simulink model "battery_phfb_inv_single_phase"  (R2024b)
settings: Solver=ode1be  StartTime=0.0  StopTime=simlength  FixedStep=ts_sim  MaxStep=ts_sim
undefined symbols (not defined in the file): Adrso, Aresd, Bresd, Cresd, Crso, dead_time, DThs_init, fPWM_INV, fPWM_ZVS, frequency_grid, I_FS, Iout_dc_nom, ki_i_inv, ki_i_zvs, ki_pll, ki_v_inv, ki_v_zvs, kp_i_inv, kp_i_zvs, kp_pll, kp_v_inv, kp_v_zvs, Ldrso, LFu_dc, magnitude, n1, number_of_cells, Q, q1kalman, q1Kalman, q2kalman, q2Kalman, q3Kalman, RCFu_dc, Rkalman, rKalman, RLFu_dc, Rload, Tambient, tc, ts_inv, ts_zvs, tsample, v1_trafo, v2_trafo, V_FS, Vout_dc_nom, w, weigth
libraries: fl_lib x207, nesl_utility x105, ee_lib x26, cstblocks x7, single_phase_transformer_lib x4, lithium_ion_cell_lib x1, simulink x1
(part 2 of 8)

== system battery_phfb_inv_single_phase/inverter_modA/single phase inverter/HBridgeIdeal ==
  gate_commands : Inport
  Bus Selector : BusSelector  OutputSignals=gate_cmd_Q1 (signal 1),gate_cmd_Q2 (signal 2),gate_cmd_Q1 (signal 3),gate_cmd_Q2 (signal 4)
  Simulink-PS Converter{,1..3} (4 alike) : nesl_utility/Simulink-PS Converter  PhysicalDomain=network_engine_domain  SubClassName=ps_input  LeftPortType=input  RightPortType=output  PseudoPeriodic=off  Frequencies=[]  NoiseDistribution=none  NoiseParameters=[]  Unit=1  AffineConversion=on  FilteringAndDerivatives=provide  SimscapeFilterOrder=1  InputFilterTimeConstant=0.001  UdotUserProvided=0
  switch_1 : Subsystem
      settings: PortSchema="{\"entries\":[{\"content\":{\"sides\":[{\"content\":{\"connectorIds\":[\"LConn1\"]},\"type\":\"ConnectorPlacement.EquallySpacedRectSide\",\"uuid\":\"9277da8d-d460-43e6-8478-dd662f15d226\"},{\"content\":{\"connectorIds\":[],\"side\":\"RIGHT\"},\"type\":\"ConnectorPlacement.EquallySpacedRectSide\",\"uuid\":\"a7ece396-f1d9-4f4f-a05b-db1fc65d6e1d\"},{\"content\":{\"connectorIds\":[\"LConn2\"],\"side\":\"TOP\"},\"type\":\"ConnectorPlacement.EquallySpacedRectSide\",\"uuid\":\"fdd70777-e9cf-4317-afb6-cae87f75d5b0\"},{\"content\":{\"connectorIds\":[\"RConn1\"],\"side\":\"BOTTOM\"},\"type\":\"ConnectorPlacement.EquallySpacedRectSide\",\"uuid\":\"2353ed68-b1a1-4775-9ca9-31e268d5443b\"}]},\"type\":\"ConnectorPlacement.EquallySpacedConnector\",\"uuid\":\"d5479f4c-4e65-4791-adcb-73df11f88590\"}],\"packageUris\":[\"http://schema.mathworks.com/mf0/Connector/R2020b\"],\"version\":\"1.0\"}"
  switch_2 : Subsystem
      settings: PortSchema="{\"entries\":[{\"content\":{\"sides\":[{\"content\":{\"connectorIds\":[\"LConn1\"]},\"type\":\"ConnectorPlacement.EquallySpacedRectSide\",\"uuid\":\"9277da8d-d460-43e6-8478-dd662f15d226\"},{\"content\":{\"connectorIds\":[],\"side\":\"RIGHT\"},\"type\":\"ConnectorPlacement.EquallySpacedRectSide\",\"uuid\":\"a7ece396-f1d9-4f4f-a05b-db1fc65d6e1d\"},{\"content\":{\"connectorIds\":[\"LConn2\"],\"side\":\"TOP\"},\"type\":\"ConnectorPlacement.EquallySpacedRectSide\",\"uuid\":\"fdd70777-e9cf-4317-afb6-cae87f75d5b0\"},{\"content\":{\"connectorIds\":[\"RConn1\"],\"side\":\"BOTTOM\"},\"type\":\"ConnectorPlacement.EquallySpacedRectSide\",\"uuid\":\"2353ed68-b1a1-4775-9ca9-31e268d5443b\"}]},\"type\":\"ConnectorPlacement.EquallySpacedConnector\",\"uuid\":\"d5479f4c-4e65-4791-adcb-73df11f88590\"}],\"packageUris\":[\"http://schema.mathworks.com/mf0/Connector/R2020b\"],\"version\":\"1.0\"}"
  switch_3 : Subsystem
      settings: PortSchema="{\"entries\":[{\"content\":{\"sides\":[{\"content\":{\"connectorIds\":[\"LConn1\"]},\"type\":\"ConnectorPlacement.EquallySpacedRectSide\",\"uuid\":\"9277da8d-d460-43e6-8478-dd662f15d226\"},{\"content\":{\"connectorIds\":[],\"side\":\"RIGHT\"},\"type\":\"ConnectorPlacement.EquallySpacedRectSide\",\"uuid\":\"a7ece396-f1d9-4f4f-a05b-db1fc65d6e1d\"},{\"content\":{\"connectorIds\":[\"LConn2\"],\"side\":\"TOP\"},\"type\":\"ConnectorPlacement.EquallySpacedRectSide\",\"uuid\":\"fdd70777-e9cf-4317-afb6-cae87f75d5b0\"},{\"content\":{\"connectorIds\":[\"RConn1\"],\"side\":\"BOTTOM\"},\"type\":\"ConnectorPlacement.EquallySpacedRectSide\",\"uuid\":\"2353ed68-b1a1-4775-9ca9-31e268d5443b\"}]},\"type\":\"ConnectorPlacement.EquallySpacedConnector\",\"uuid\":\"d5479f4c-4e65-4791-adcb-73df11f88590\"}],\"packageUris\":[\"http://schema.mathworks.com/mf0/Connector/R2020b\"],\"version\":\"1.0\"}"
  switch_4 : Subsystem
      settings: PortSchema="{\"entries\":[{\"content\":{\"sides\":[{\"content\":{\"connectorIds\":[\"LConn1\"]},\"type\":\"ConnectorPlacement.EquallySpacedRectSide\",\"uuid\":\"9277da8d-d460-43e6-8478-dd662f15d226\"},{\"content\":{\"connectorIds\":[],\"side\":\"RIGHT\"},\"type\":\"ConnectorPlacement.EquallySpacedRectSide\",\"uuid\":\"a7ece396-f1d9-4f4f-a05b-db1fc65d6e1d\"},{\"content\":{\"connectorIds\":[\"LConn2\"],\"side\":\"TOP\"},\"type\":\"ConnectorPlacement.EquallySpacedRectSide\",\"uuid\":\"fdd70777-e9cf-4317-afb6-cae87f75d5b0\"},{\"content\":{\"connectorIds\":[\"RConn1\"],\"side\":\"BOTTOM\"},\"type\":\"ConnectorPlacement.EquallySpacedRectSide\",\"uuid\":\"2353ed68-b1a1-4775-9ca9-31e268d5443b\"}]},\"type\":\"ConnectorPlacement.EquallySpacedConnector\",\"uuid\":\"d5479f4c-4e65-4791-adcb-73df11f88590\"}],\"packageUris\":[\"http://schema.mathworks.com/mf0/Connector/R2020b\"],\"version\":\"1.0\"}"
  C : PMIOPort  Side=Left
  E : PMIOPort  Port=2  Side=Right
  C1 : PMIOPort  Port=3  Side=Right
  E1 : PMIOPort  Port=4  Side=Left
  wires:
  [gate_Q3] -> Simulink-PS Converter2/1
  Bus Selector/2 -> [gate_Q2]  "<gate_cmd_Q2 (signal 2)>"
  Bus Selector/1 -> [gate_Q1]  "<gate_cmd_Q1 (signal 1)>"
  Bus Selector/3 -> [gate_Q3]  "<gate_cmd_Q1 (signal 3)>"
  [gate_Q4] -> Simulink-PS Converter3/1
  [gate_Q2] -> Simulink-PS Converter1/1
  [gate_Q1] -> Simulink-PS Converter/1
  Bus Selector/4 -> [gate_Q4]  "<gate_cmd_Q2 (signal 4)>"
  gate_commands/1 -> Bus Selector/1
  connections:
  switch_1/LConn1 -- Simulink-PS Converter/RConn1
  switch_3/LConn2 -- C/RConn1 -- switch_1/LConn2
  switch_4/RConn1 -- E1/RConn1 -- switch_2/RConn1
  switch_2/LConn2 -- E/RConn1 -- switch_1/RConn1
  switch_3/LConn1 -- Simulink-PS Converter2/RConn1
  switch_3/RConn1 -- C1/RConn1 -- switch_4/LConn2
  switch_2/LConn1 -- Simulink-PS Converter1/RConn1
  switch_4/LConn1 -- Simulink-PS Converter3/RConn1

== system battery_phfb_inv_single_phase/inverter_modA/single phase inverter/HBridgeMosfet ==
  gate_commands : Inport
  Bus Selector : BusSelector  OutputSignals=gate_cmd_Q1,gate_cmd_Q2,gate_cmd_Q3,gate_cmd_Q4
  Simulink-PS Converter{,1..3} (4 alike) : nesl_utility/Simulink-PS Converter  PhysicalDomain=network_engine_domain  SubClassName=ps_input  LeftPortType=input  RightPortType=output  PseudoPeriodic=off  Frequencies=[]  NoiseDistribution=none  NoiseParameters=[]  Unit=V  AffineConversion=off  FilteringAndDerivatives=provide  SimscapeFilterOrder=1  InputFilterTimeConstant=0.001  UdotUserProvided=0
  mosfet_1 : Subsystem
      settings: PortSchema="{\"entries\":[{\"content\":{\"sides\":[{\"content\":{\"connectorIds\":[\"LConn1\"]},\"type\":\"ConnectorPlacement.EquallySpacedRectSide\",\"uuid\":\"9277da8d-d460-43e6-8478-dd662f15d226\"},{\"content\":{\"connectorIds\":[],\"side\":\"RIGHT\"},\"type\":\"ConnectorPlacement.EquallySpacedRectSide\",\"uuid\":\"a7ece396-f1d9-4f4f-a05b-db1fc65d6e1d\"},{\"content\":{\"connectorIds\":[\"LConn2\"],\"side\":\"TOP\"},\"type\":\"ConnectorPlacement.EquallySpacedRectSide\",\"uuid\":\"fdd70777-e9cf-4317-afb6-cae87f75d5b0\"},{\"content\":{\"connectorIds\":[\"RConn1\"],\"side\":\"BOTTOM\"},\"type\":\"ConnectorPlacement.EquallySpacedRectSide\",\"uuid\":\"2353ed68-b1a1-4775-9ca9-31e268d5443b\"}]},\"type\":\"ConnectorPlacement.EquallySpacedConnector\",\"uuid\":\"d5479f4c-4e65-4791-adcb-73df11f88590\"}],\"packageUris\":[\"http://schema.mathworks.com/mf0/Connector/R2020b\"],\"version\":\"1.0\"}"
  mosfet_2 : Subsystem
      settings: PortSchema="{\"entries\":[{\"content\":{\"sides\":[{\"content\":{\"connectorIds\":[\"LConn1\"]},\"type\":\"ConnectorPlacement.EquallySpacedRectSide\",\"uuid\":\"9277da8d-d460-43e6-8478-dd662f15d226\"},{\"content\":{\"connectorIds\":[],\"side\":\"RIGHT\"},\"type\":\"ConnectorPlacement.EquallySpacedRectSide\",\"uuid\":\"a7ece396-f1d9-4f4f-a05b-db1fc65d6e1d\"},{\"content\":{\"connectorIds\":[\"LConn2\"],\"side\":\"TOP\"},\"type\":\"ConnectorPlacement.EquallySpacedRectSide\",\"uuid\":\"fdd70777-e9cf-4317-afb6-cae87f75d5b0\"},{\"content\":{\"connectorIds\":[\"RConn1\"],\"side\":\"BOTTOM\"},\"type\":\"ConnectorPlacement.EquallySpacedRectSide\",\"uuid\":\"2353ed68-b1a1-4775-9ca9-31e268d5443b\"}]},\"type\":\"ConnectorPlacement.EquallySpacedConnector\",\"uuid\":\"d5479f4c-4e65-4791-adcb-73df11f88590\"}],\"packageUris\":[\"http://schema.mathworks.com/mf0/Connector/R2020b\"],\"version\":\"1.0\"}"
  mosfet_3 : Subsystem
      settings: PortSchema="{\"entries\":[{\"content\":{\"sides\":[{\"content\":{\"connectorIds\":[\"LConn1\"]},\"type\":\"ConnectorPlacement.EquallySpacedRectSide\",\"uuid\":\"9277da8d-d460-43e6-8478-dd662f15d226\"},{\"content\":{\"connectorIds\":[],\"side\":\"RIGHT\"},\"type\":\"ConnectorPlacement.EquallySpacedRectSide\",\"uuid\":\"a7ece396-f1d9-4f4f-a05b-db1fc65d6e1d\"},{\"content\":{\"connectorIds\":[\"LConn2\"],\"side\":\"TOP\"},\"type\":\"ConnectorPlacement.EquallySpacedRectSide\",\"uuid\":\"fdd70777-e9cf-4317-afb6-cae87f75d5b0\"},{\"content\":{\"connectorIds\":[\"RConn1\"],\"side\":\"BOTTOM\"},\"type\":\"ConnectorPlacement.EquallySpacedRectSide\",\"uuid\":\"2353ed68-b1a1-4775-9ca9-31e268d5443b\"}]},\"type\":\"ConnectorPlacement.EquallySpacedConnector\",\"uuid\":\"d5479f4c-4e65-4791-adcb-73df11f88590\"}],\"packageUris\":[\"http://schema.mathworks.com/mf0/Connector/R2020b\"],\"version\":\"1.0\"}"
  mosfet_4 : Subsystem
      settings: PortSchema="{\"entries\":[{\"content\":{\"sides\":[{\"content\":{\"connectorIds\":[\"LConn1\"]},\"type\":\"ConnectorPlacement.EquallySpacedRectSide\",\"uuid\":\"9277da8d-d460-43e6-8478-dd662f15d226\"},{\"content\":{\"connectorIds\":[],\"side\":\"RIGHT\"},\"type\":\"ConnectorPlacement.EquallySpacedRectSide\",\"uuid\":\"a7ece396-f1d9-4f4f-a05b-db1fc65d6e1d\"},{\"content\":{\"connectorIds\":[\"LConn2\"],\"side\":\"TOP\"},\"type\":\"ConnectorPlacement.EquallySpacedRectSide\",\"uuid\":\"fdd70777-e9cf-4317-afb6-cae87f75d5b0\"},{\"content\":{\"connectorIds\":[\"RConn1\"],\"side\":\"BOTTOM\"},\"type\":\"ConnectorPlacement.EquallySpacedRectSide\",\"uuid\":\"2353ed68-b1a1-4775-9ca9-31e268d5443b\"}]},\"type\":\"ConnectorPlacement.EquallySpacedConnector\",\"uuid\":\"d5479f4c-4e65-4791-adcb-73df11f88590\"}],\"packageUris\":[\"http://schema.mathworks.com/mf0/Connector/R2020b\"],\"version\":\"1.0\"}"
  C : PMIOPort  Side=Left
  E : PMIOPort  Port=2  Side=Right
  C1 : PMIOPort  Port=3  Side=Right
  E1 : PMIOPort  Port=4  Side=Left
  wires:
  [gate_Q3] -> Simulink-PS Converter2/1
  Bus Selector/2 -> [gate_Q2]  "<gate_cmd_Q2>"
  Bus Selector/1 -> [gate_Q1]  "<gate_cmd_Q1>"
  Bus Selector/3 -> [gate_Q3]  "<gate_cmd_Q3>"
  [gate_Q4] -> Simulink-PS Converter3/1
  [gate_Q2] -> Simulink-PS Converter1/1
  [gate_Q1] -> Simulink-PS Converter/1
  Bus Selector/4 -> [gate_Q4]  "<gate_cmd_Q4>"
  gate_commands/1 -> Bus Selector/1
  connections:
  mosfet_1/LConn1 -- Simulink-PS Converter/RConn1
  C/RConn1 -- mosfet_3/LConn2 -- mosfet_1/LConn2
  E1/RConn1 -- mosfet_4/RConn1 -- mosfet_2/RConn1
  E/RConn1 -- mosfet_2/LConn2 -- mosfet_1/RConn1
  mosfet_3/LConn1 -- Simulink-PS Converter2/RConn1
  C1/RConn1 -- mosfet_4/LConn2 -- mosfet_3/RConn1
  mosfet_2/LConn1 -- Simulink-PS Converter1/RConn1
  mosfet_4/LConn1 -- Simulink-PS Converter3/RConn1

== system battery_phfb_inv_single_phase/inverter_modA/single phase inverter/HBridgeThermal ==
  gate_commands : Inport
  Bus Selector : BusSelector  OutputSignals=gate_cmd_Q1,gate_cmd_Q2,gate_cmd_Q3,gate_cmd_Q4
  Simulink-PS Converter{,1..3} (4 alike) : nesl_utility/Simulink-PS Converter  PhysicalDomain=network_engine_domain  SubClassName=ps_input  LeftPortType=input  RightPortType=output  PseudoPeriodic=off  Frequencies=[]  NoiseDistribution=none  NoiseParameters=[]  Unit=V  AffineConversion=off  FilteringAndDerivatives=provide  SimscapeFilterOrder=1  InputFilterTimeConstant=0.001  UdotUserProvided=0
  mosfet_thermal_1 : Subsystem
      settings: PortSchema="{\"entries\":[{\"content\":{\"sides\":[{\"content\":{\"connectorIds\":[\"LConn1\"]},\"type\":\"ConnectorPlacement.EquallySpacedRectSide\",\"uuid\":\"9277da8d-d460-43e6-8478-dd662f15d226\"},{\"content\":{\"connectorIds\":[],\"side\":\"RIGHT\"},\"type\":\"ConnectorPlacement.EquallySpacedRectSide\",\"uuid\":\"a7ece396-f1d9-4f4f-a05b-db1fc65d6e1d\"},{\"content\":{\"connectorIds\":[\"LConn2\"],\"side\":\"TOP\"},\"type\":\"ConnectorPlacement.EquallySpacedRectSide\",\"uuid\":\"fdd70777-e9cf-4317-afb6-cae87f75d5b0\"},{\"content\":{\"connectorIds\":[\"RConn1\"],\"side\":\"BOTTOM\"},\"type\":\"ConnectorPlacement.EquallySpacedRectSide\",\"uuid\":\"2353ed68-b1a1-4775-9ca9-31e268d5443b\"}]},\"type\":\"ConnectorPlacement.EquallySpacedConnector\",\"uuid\":\"d5479f4c-4e65-4791-adcb-73df11f88590\"}],\"packageUris\":[\"http://schema.mathworks.com/mf0/Connector/R2020b\"],\"version\":\"1.0\"}"
  mosfet_thermal_2 : Subsystem
      settings: PortSchema="{\"entries\":[{\"content\":{\"sides\":[{\"content\":{\"connectorIds\":[\"LConn1\"]},\"type\":\"ConnectorPlacement.EquallySpacedRectSide\",\"uuid\":\"9277da8d-d460-43e6-8478-dd662f15d226\"},{\"content\":{\"connectorIds\":[],\"side\":\"RIGHT\"},\"type\":\"ConnectorPlacement.EquallySpacedRectSide\",\"uuid\":\"a7ece396-f1d9-4f4f-a05b-db1fc65d6e1d\"},{\"content\":{\"connectorIds\":[\"LConn2\"],\"side\":\"TOP\"},\"type\":\"ConnectorPlacement.EquallySpacedRectSide\",\"uuid\":\"fdd70777-e9cf-4317-afb6-cae87f75d5b0\"},{\"content\":{\"connectorIds\":[\"RConn1\"],\"side\":\"BOTTOM\"},\"type\":\"ConnectorPlacement.EquallySpacedRectSide\",\"uuid\":\"2353ed68-b1a1-4775-9ca9-31e268d5443b\"}]},\"type\":\"ConnectorPlacement.EquallySpacedConnector\",\"uuid\":\"d5479f4c-4e65-4791-adcb-73df11f88590\"}],\"packageUris\":[\"http://schema.mathworks.com/mf0/Connector/R2020b\"],\"version\":\"1.0\"}"
  mosfet_thermal_3 : Subsystem
      settings: PortSchema="{\"entries\":[{\"content\":{\"sides\":[{\"content\":{\"connectorIds\":[\"LConn1\"]},\"type\":\"ConnectorPlacement.EquallySpacedRectSide\",\"uuid\":\"9277da8d-d460-43e6-8478-dd662f15d226\"},{\"content\":{\"connectorIds\":[],\"side\":\"RIGHT\"},\"type\":\"ConnectorPlacement.EquallySpacedRectSide\",\"uuid\":\"a7ece396-f1d9-4f4f-a05b-db1fc65d6e1d\"},{\"content\":{\"connectorIds\":[\"LConn2\"],\"side\":\"TOP\"},\"type\":\"ConnectorPlacement.EquallySpacedRectSide\",\"uuid\":\"fdd70777-e9cf-4317-afb6-cae87f75d5b0\"},{\"content\":{\"connectorIds\":[\"RConn1\"],\"side\":\"BOTTOM\"},\"type\":\"ConnectorPlacement.EquallySpacedRectSide\",\"uuid\":\"2353ed68-b1a1-4775-9ca9-31e268d5443b\"}]},\"type\":\"ConnectorPlacement.EquallySpacedConnector\",\"uuid\":\"d5479f4c-4e65-4791-adcb-73df11f88590\"}],\"packageUris\":[\"http://schema.mathworks.com/mf0/Connector/R2020b\"],\"version\":\"1.0\"}"
  mosfet_thermal_4 : Subsystem
      settings: PortSchema="{\"entries\":[{\"content\":{\"sides\":[{\"content\":{\"connectorIds\":[\"LConn1\"]},\"type\":\"ConnectorPlacement.EquallySpacedRectSide\",\"uuid\":\"9277da8d-d460-43e6-8478-dd662f15d226\"},{\"content\":{\"connectorIds\":[],\"side\":\"RIGHT\"},\"type\":\"ConnectorPlacement.EquallySpacedRectSide\",\"uuid\":\"a7ece396-f1d9-4f4f-a05b-db1fc65d6e1d\"},{\"content\":{\"connectorIds\":[\"LConn2\"],\"side\":\"TOP\"},\"type\":\"ConnectorPlacement.EquallySpacedRectSide\",\"uuid\":\"fdd70777-e9cf-4317-afb6-cae87f75d5b0\"},{\"content\":{\"connectorIds\":[\"RConn1\"],\"side\":\"BOTTOM\"},\"type\":\"ConnectorPlacement.EquallySpacedRectSide\",\"uuid\":\"2353ed68-b1a1-4775-9ca9-31e268d5443b\"}]},\"type\":\"ConnectorPlacement.EquallySpacedConnector\",\"uuid\":\"d5479f4c-4e65-4791-adcb-73df11f88590\"}],\"packageUris\":[\"http://schema.mathworks.com/mf0/Connector/R2020b\"],\"version\":\"1.0\"}"
  C : PMIOPort  Side=Left
  E : PMIOPort  Port=2  Side=Right
  C1 : PMIOPort  Port=3  Side=Right
  E1 : PMIOPort  Port=4  Side=Left
  wires:
  gate_commands/1 -> Bus Selector/1
  Bus Selector/4 -> [gate_Q4]  "<gate_cmd_Q4>"
  [gate_Q1] -> Simulink-PS Converter/1
  [gate_Q2] -> Simulink-PS Converter1/1
  [gate_Q4] -> Simulink-PS Converter3/1
  Bus Selector/3 -> [gate_Q3]  "<gate_cmd_Q3>"
  Bus Selector/1 -> [gate_Q1]  "<gate_cmd_Q1>"
  Bus Selector/2 -> [gate_Q2]  "<gate_cmd_Q2>"
  [gate_Q3] -> Simulink-PS Converter2/1
  connections:
  mosfet_thermal_4/LConn1 -- Simulink-PS Converter3/RConn1
  mosfet_thermal_2/LConn1 -- Simulink-PS Converter1/RConn1
  C1/RConn1 -- mosfet_thermal_4/LConn2 -- mosfet_thermal_3/RConn1
  mosfet_thermal_3/LConn1 -- Simulink-PS Converter2/RConn1
  E/RConn1 -- mosfet_thermal_1/RConn1 -- mosfet_thermal_2/LConn2
  E1/RConn1 -- mosfet_thermal_4/RConn1 -- mosfet_thermal_2/RConn1
  mosfet_thermal_1/LConn2 -- mosfet_thermal_3/LConn2 -- C/RConn1
  mosfet_thermal_1/LConn1 -- Simulink-PS Converter/RConn1

== system battery_phfb_inv_single_phase/inverter_modA/single phase inverter control/acquisition_and_scaling_current ==
  in : Inport
  1/Ti5 : Gain  Gain=1/I_FS  SaturateOnIntegerOverflow=on  OutDataTypeStr=Inherit: Same as input  ParamDataTypeStr=Inherit: Same as input
  Unit Delay4 : UnitDelay  SampleTime=ts_inv  HasFrameUpgradeWarning=on
  Zero-Order Hold1 : ZeroOrderHold  SampleTime=ts_inv
  out : Outport
  wires:
  in/1 -> Zero-Order Hold1/1
  1/Ti5/1 -> Unit Delay4/1
  Zero-Order Hold1/1 -> 1/Ti5/1
  Unit Delay4/1 -> out/1

== system battery_phfb_inv_single_phase/inverter_modA/single phase inverter control/acquisition_and_scaling_voltage ==
  in : Inport
  1/Ti1 : Gain  Gain=1/V_FS  SaturateOnIntegerOverflow=on  OutDataTypeStr=Inherit: Same as input  ParamDataTypeStr=Inherit: Same as input
  Unit Delay4 : UnitDelay  SampleTime=ts_inv  HasFrameUpgradeWarning=on
  Zero-Order Hold2 : ZeroOrderHold  SampleTime=ts_inv
  out : Outport
  wires:
  1/Ti1/1 -> Unit Delay4/1
  Zero-Order Hold2/1 -> 1/Ti1/1
  Unit Delay4/1 -> out/1
  in/1 -> Zero-Order Hold2/1

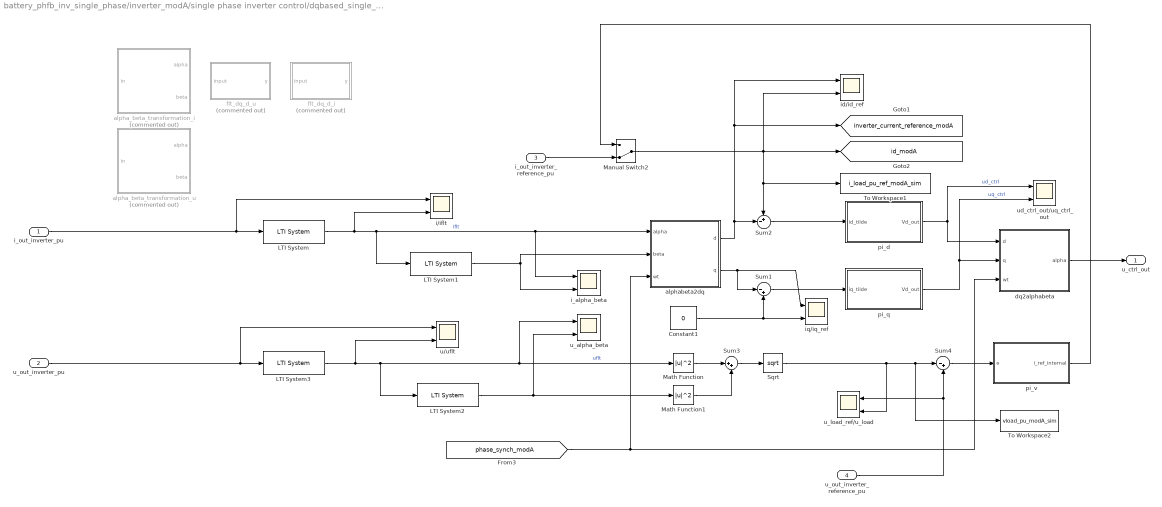
== system battery_phfb_inv_single_phase/inverter_modA/single phase inverter control/dqbased_single_phase_inverter_ctrl ==
  i_out_inverter_pu : Inport
  u_out_inverter_pu : Inport  Port=2
  i_out_inverter_reference_pu : Inport  Port=3
  u_out_inverter_reference_pu : Inport  Port=4
  Constant1 : Constant  Value=0
  LTI System : cstblocks/LTI System  sys=resd_tf  IC=[]  PadeOrder=0
  LTI System1 : cstblocks/LTI System  sys=flt_dq_d  IC=[]  PadeOrder=0
  LTI System2 : cstblocks/LTI System  sys=flt_dq_d  IC=[]  PadeOrder=0
  LTI System3 : cstblocks/LTI System  sys=resd_tf  IC=[]  PadeOrder=0
  Manual Switch2 : ManualSwitch  CurrentSetting=0
  Math Function : Math  Operator=magnitude^2
  Math Function1 : Math  Operator=magnitude^2
  Sqrt : Sqrt
  Sum1 : Sum  Inputs=|-+
  Sum2 : Sum  Inputs=+-|
  Sum3 : Sum  Inputs=|++
  Sum4 : Sum  Inputs=|-+
  To Workspace1 : ToWorkspace  VariableName=i_load_pu_ref_modA_sim  SampleTime=ts_inv
      settings: MaxDataPoints=Ns_inv
  To Workspace2 : ToWorkspace  VariableName=vload_pu_modA_sim  SampleTime=ts_inv
      settings: MaxDataPoints=Ns_inv
  alpha_beta_transformation_i : Subsystem  Commented=on
  alpha_beta_transformation_u : Subsystem  Commented=on
  alphabeta2dq : Subsystem
  dq2alphabeta : Subsystem
  flt_dq_d_i : MATLAB Function  Commented=on  TreatAsAtomicUnit=on  SystemSampleTime=ts_inv
  flt_dq_d_u : MATLAB Function  Commented=on  TreatAsAtomicUnit=on  SystemSampleTime=ts_inv
  i/iflt : Scope  NumInputPorts=2
  i_alpha_beta : Scope  NumInputPorts=2
  id/id_ref : Scope  NumInputPorts=2
  iq/iq_ref : Scope  NumInputPorts=2
  pi_d : Subsystem
  pi_q : Subsystem
  pi_v : Subsystem
  u/uflt : Scope  NumInputPorts=2
  u_alpha_beta : Scope  NumInputPorts=2
  u_load_ref/u_load : Scope  NumInputPorts=2
  ud_ctrl_out/uq_ctrl_out : Scope  NumInputPorts=2
  u_ctrl_out : Outport
  tag scope: id_modA=global, inverter_current_reference_modA=global
  wires:
  alphabeta2dq/1("d ") -> Sum2/2, id/id_ref/1, [inverter_current_reference_modA]
  Sqrt/1 -> u_load_ref/u_load/2, To Workspace2/1, Sum4/1
  i_out_inverter_pu/1 -> LTI System/1, i/iflt/1
  Math Function/1 -> Sum3/1
  LTI System1/1 -> alphabeta2dq/2(beta), i_alpha_beta/2
  LTI System/1 -> i/iflt/2, LTI System1/1, alphabeta2dq/1(alpha), i_alpha_beta/1  "iflt"
  [phase_synch_modA] -> alphabeta2dq/3(wt), dq2alphabeta/3(wt)
  pi_q/1(Vd_out) -> dq2alphabeta/2(q), ud_ctrl_out/uq_ctrl_out/2  "uq_ctrl"
  alphabeta2dq/2("q ") -> Sum1/1, iq/iq_ref/1
  Sum4/1 -> pi_v/1(e)
  pi_d/1(Vd_out) -> ud_ctrl_out/uq_ctrl_out/1, dq2alphabeta/1(d)  "ud_ctrl"
  Manual Switch2/1 -> id/id_ref/2, [id_modA], Sum2/1, To Workspace1/1
  i_out_inverter_reference_pu/1 -> Manual Switch2/2
  LTI System3/1 -> Math Function/1, u_alpha_beta/1, LTI System2/1, u/uflt/2  "uflt"
  Sum1/1 -> pi_q/1(iq_tilde)
  Math Function1/1 -> Sum3/2
  Sum2/1 -> pi_d/1(id_tilde)
  LTI System2/1 -> u_alpha_beta/2, Math Function1/1
  Constant1/1 -> iq/iq_ref/2, Sum1/2
  u_out_inverter_pu/1 -> LTI System3/1, u/uflt/1
  pi_v/1(i_ref_internal) -> Manual Switch2/1
  dq2alphabeta/1(alpha) -> u_ctrl_out/1
  Sum3/1 -> Sqrt/1
  u_out_inverter_reference_pu/1 -> u_load_ref/u_load/1, Sum4/2

== system battery_phfb_inv_single_phase/inverter_modA/single phase inverter control/pwm ==
  vout : Inport
  Constant : Constant  Value=0
  Constant{1..4} (4 alike) : Constant
  Gain1 : Gain  Gain=1/2
  Gain2 : Gain
  Gain3 : Gain  Gain=1/2
  Gain4 : Gain  Gain=-1
  PWM generator 1 : Subsystem  mask{f=fPWM_INV, m_up=0.98, m_low=0.02, dead_time=dead_time, pos_cmd_gate=15, neg_cmd_gate=-10, polarity=-1}
      mask prompts: f "Frequency (Hz)"; m_up "Max Input Modulation Value"; m_low "Min Input Modulation Value"; dead_time "Dead Time (s)"; pos_cmd_gate "Positive Gate Voltage (V)"; neg_cmd_gate "Negative Gate Voltage (V)"; polarity "Polarity (pu)"
  PWM generator 2 : Subsystem  mask{f=fPWM_INV, m_up=0.98, m_low=0.02, dead_time=dead_time, pos_cmd_gate=15, neg_cmd_gate=-10, polarity=-1}
      mask prompts: f "Frequency (Hz)"; m_up "Max Input Modulation Value"; m_low "Min Input Modulation Value"; dead_time "Dead Time (s)"; pos_cmd_gate "Positive Gate Voltage (V)"; neg_cmd_gate "Negative Gate Voltage (V)"; polarity "Polarity (pu)"
  Product{,1..3} (4 alike) : Product
  Sum : Sum  Inputs=|++
  Sum1 : Sum  Inputs=|++
  m1_top : Outport
  m1_bottom : Outport  Port=2
  m2_top : Outport  Port=3
  m2_bottom : Outport  Port=4
  wires:
  Constant/1 -> PWM generator 2/2(phase), PWM generator 1/2(phase)
  Constant1/1 -> PWM generator 2/3(polarity_input), PWM generator 1/3(polarity_input)
  Gain2/1 -> Sum/1
  Sum/1 -> Gain1/1
  Constant2/1 -> Sum/2
  Gain1/1 -> PWM generator 1/1(m_index)
  Constant3/1 -> Sum1/2
  Sum1/1 -> Gain3/1
  Gain4/1 -> Sum1/1
  Gain3/1 -> PWM generator 2/1(m_index)
  vout/1 -> Gain4/1, Gain2/1
  PWM generator 1/1(m1) -> Product/1  "gate_cmd_Q1"
  PWM generator 1/2(m2) -> Product1/1  "gate_cmd_Q2"
  PWM generator 2/1(m1) -> Product2/1  "gate_cmd_Q3"
  PWM generator 2/2(m2) -> Product3/1  "gate_cmd_Q4"
  Product/1 -> m1_top/1  "gate_cmd_Q1"
  Product1/1 -> m1_bottom/1  "gate_cmd_Q2"
  Product2/1 -> m2_top/1  "gate_cmd_Q3"
  Product3/1 -> m2_bottom/1  "gate_cmd_Q4"
  Constant4/1 -> Product3/2, Product2/2, Product1/2, Product/2

== system battery_phfb_inv_single_phase/inverter_modA/single phase inverter control/references_generator ==
  1/Ti2 : Gain  Gain=1/V_FS  SaturateOnIntegerOverflow=on  OutDataTypeStr=Inherit: Same as input  ParamDataTypeStr=Inherit: Same as input
  1/Ti4 : Gain  Gain=1/I_FS  SaturateOnIntegerOverflow=on  OutDataTypeStr=Inherit: Same as input  ParamDataTypeStr=Inherit: Same as input
  Rate Limiter : RateLimiter  SampleTimeMode=inherited
  Rate Limiter1 : RateLimiter  SampleTimeMode=inherited
  Zero-Order Hold3 : ZeroOrderHold  SampleTime=ts_inv
  Zero-Order Hold4 : ZeroOrderHold  SampleTime=ts_inv
  i_out_inverter_reference : Step  Time=0.75  After=-I_FS  SampleTime=0
  u_out_inverter_reference : Step  Time=0.5  After=230*sqrt(2)  SampleTime=0
  i_out_inverter_reference_pu : Outport
  u_out_inverter_reference_pu : Outport  Port=2
  wires:
  Zero-Order Hold3/1 -> i_out_inverter_reference_pu/1
  1/Ti4/1 -> Rate Limiter1/1
  1/Ti2/1 -> Rate Limiter/1
  Rate Limiter/1 -> Zero-Order Hold4/1
  Zero-Order Hold4/1 -> u_out_inverter_reference_pu/1
  Rate Limiter1/1 -> Zero-Order Hold3/1
  i_out_inverter_reference/1 -> 1/Ti4/1
  u_out_inverter_reference/1 -> 1/Ti2/1

== system battery_phfb_inv_single_phase/inverter_modA/single phase inverter control/rpi_based_single_phase_inverter_ctrl ==
  i_out_inverter_pu : Inport
  u_out_inverter_pu : Inport  Port=2
  i_out_inverter_reference_pu : Inport  Port=3
  u_out_inverter_reference_pu : Inport  Port=4
  Manual Switch2 : ManualSwitch
  current_reference_generation : Subsystem
  is/is_ref : Scope  NumInputPorts=2
  load_current_control : Subsystem
  load_voltage_control : Subsystem
  u_ctrl_out : Outport
  tag scope: i_out_inverter_pu=global, i_out_inverter_pu_ref=global, id_inv_pu_ref=global
  wires:
  i_out_inverter_pu/1 -> load_current_control/2(i_out_inverter_pu), [i_out_inverter_pu], is/is_ref/1  "i_out_inverter_pu"
  load_current_control/1(u_ctrl_out) -> u_ctrl_out/1  "u_ctrl_out"
  current_reference_generation/1(phase_ref) -> [i_out_inverter_pu_ref], is/is_ref/2, load_current_control/1(i_out_inverter_reference_pu)  "i_out_inverter_pu_ref"
  Manual Switch2/1 -> [id_inv_pu_ref], current_reference_generation/1(mag_ref)
  i_out_inverter_reference_pu/1 -> Manual Switch2/2
  u_out_inverter_pu/1 -> load_voltage_control/1(u_load)  "u_out_inverter_pu"
  u_out_inverter_reference_pu/1 -> load_voltage_control/2(u_load_reference)  "u_out_inverter_reference_pu"
  load_voltage_control/1(i_ref_internal) -> Manual Switch2/1

== system battery_phfb_inv_single_phase/inverter_modA/single_phase_pll/double_integrator_observer ==
  theta : Inport
  Gain : Gain  Gain=Ldrso  Multiplication=Matrix(K*u)
  Gain1 : Gain  Gain=Adrso  Multiplication=Matrix(K*u)
  Gain2 : Gain  Gain=Crso  Multiplication=Matrix(K*u)
  Sum : Sum  Inputs=-+|
  Sum1 : Sum  Inputs=|++
  Unit Delay : UnitDelay  SampleTime=ts_inv  HasFrameUpgradeWarning=on
  Zero-Order Hold : ZeroOrderHold  SampleTime=ts_inv
  bounder1 : MATLAB Function  TreatAsAtomicUnit=on  SystemSampleTime=ts_inv
  bounder2 : MATLAB Function  TreatAsAtomicUnit=on  SystemSampleTime=ts_inv
  theta_hat : Outport
  wires:
  Gain/1 -> Sum1/1
  Gain2/1 -> bounder2/1(u)  "theta_hat"
  Gain1/1 -> Sum1/2
  Sum1/1 -> Unit Delay/1
  Sum/1 -> bounder1/1(u)  "e"
  Unit Delay/1 -> Gain1/1, Gain2/1
  theta/1 -> Zero-Order Hold/1  "theta"
  Zero-Order Hold/1 -> Sum/2  "theta_dsp"
  bounder1/1(y) -> Gain/1  "e_bounded"
  bounder2/1(y) -> theta_hat/1, Sum/1  "theta_hat_bounded"

== system battery_phfb_inv_single_phase/inverter_modA/single_phase_pll/pi-ctrl ==
  x : Inport
  xref : Inport  Port=2
  1/Ti : Gain  Gain=kp  SaturateOnIntegerOverflow=on  OutDataTypeStr=Inherit: Same as input  ParamDataTypeStr=Inherit: Same as input
  Saturation : Saturate  UpperLimit=sat_pos  LowerLimit=sat_neg
  Sum1 : Sum  Inputs=+++  SaturateOnIntegerOverflow=on
  Sum2 : Sum  Inputs=-+  SaturateOnIntegerOverflow=on
  Sum3 : Sum  Inputs=-+  SaturateOnIntegerOverflow=on
  Unit Delay1 : UnitDelay  SampleTime=ts  HasFrameUpgradeWarning=on
  Unit Delay2 : UnitDelay  SampleTime=ts  HasFrameUpgradeWarning=on
  Unit Delay4 : UnitDelay  SampleTime=ts  HasFrameUpgradeWarning=on
  kp : Gain  Gain=ki*ts  SaturateOnIntegerOverflow=on  OutDataTypeStr=Inherit: Same as input  ParamDataTypeStr=Inherit: Same as input
  u : Outport
  wires:
  Saturation/1 -> Sum3/2, u/1
  Unit Delay4/1 -> Sum1/3
  Sum1/1 -> Saturation/1
  x/1 -> Unit Delay1/1
  Sum3/1 -> Unit Delay4/1
  1/Ti/1 -> Sum3/1, Sum1/1
  Sum2/1 -> 1/Ti/1, kp/1
  kp/1 -> Sum1/2
  xref/1 -> Unit Delay2/1
  Unit Delay1/1 -> Sum2/1
  Unit Delay2/1 -> Sum2/2

== system battery_phfb_inv_single_phase/zvs_modA/battery_system/LithiumIonBattery ==
  Current Sensor : fl_lib/Electrical/Electrical Sensors/Current Sensor
  Electrical Reference1 : fl_lib/Electrical/Electrical Elements/Electrical Reference
  PS-Simulink Converter4 : nesl_utility/PS-Simulink Converter  PhysicalDomain=network_engine_domain  SubClassName=ps_output  LeftPortType=input  RightPortType=output  PseudoPeriodic=off  Frequencies=[]  VectorFormat=1-D array  Unit=1  AffineConversion=off
  PS-Simulink Converter5 : nesl_utility/PS-Simulink Converter  PhysicalDomain=network_engine_domain  SubClassName=ps_output  LeftPortType=input  RightPortType=output  PseudoPeriodic=off  Frequencies=[]  VectorFormat=1-D array  Unit=V  AffineConversion=on
  SOC_estimator : Subsystem
  To Workspace1 : ToWorkspace  VariableName=idc_battery_sim  SampleTime=tc
      settings: MaxDataPoints=Nc
  To Workspace2 : ToWorkspace  VariableName=udc_battery_sim  SampleTime=tc
      settings: MaxDataPoints=Nc
  Unit Delay5 : UnitDelay  SampleTime=ts_zvs  HasFrameUpgradeWarning=on
  Voltage Sensor : fl_lib/Electrical/Electrical Sensors/Voltage Sensor
  ibat/vdc : Scope  NumInputPorts=2
  lithium ion cell analytical ocv : Subsystem
  Uout+ : PMIOPort  Side=Right
  Uout- : PMIOPort  Port=2  Side=Right
  wires:
  PS-Simulink Converter5/1 -> Unit Delay5/1
  PS-Simulink Converter4/1 -> To Workspace1/1, ibat/vdc/1  "i batt"
  Unit Delay5/1 -> To Workspace2/1, [vdc]
  [vdc] -> ibat/vdc/2  "vdc"
  connections:
  Current Sensor/RConn1 -- PS-Simulink Converter4/LConn1
  Uout+/RConn1 -- Current Sensor/RConn2 -- Voltage Sensor/LConn1
  Voltage Sensor/RConn1 -- PS-Simulink Converter5/LConn1
  Voltage Sensor/RConn2 -- Electrical Reference1/LConn1 -- lithium ion cell analytical ocv/RConn2 -- Uout-/RConn1
  lithium ion cell analytical ocv/RConn1 -- Current Sensor/LConn1

== system battery_phfb_inv_single_phase/zvs_modA/dc//dc with galvanic isolation/stage-1 ==
  gate_commands : Inport
  Current Sensor : fl_lib/Electrical/Electrical Sensors/Current Sensor
  PS-Simulink Converter1 : nesl_utility/PS-Simulink Converter  PhysicalDomain=network_engine_domain  SubClassName=ps_output  LeftPortType=input  RightPortType=output  PseudoPeriodic=off  Frequencies=[]  VectorFormat=1-D array  Unit=A  AffineConversion=on
  h-bridge_thermal : Subsystem  Commented=on
  h-ideal : Subsystem  Commented=on
  h-mosfet : Subsystem
  uac_1(+) : PMIOPort  Side=Left
  uac_1(-) : PMIOPort  Port=2  Side=Left
  Udc(+) : PMIOPort  Port=3  Side=Right
  Udc(-) : PMIOPort  Port=4  Side=Right
  tag scope: dc_bus_terminal_current_inverter=global
  wires:
  gate_commands/1 -> h-mosfet/1(gate_commands)
  PS-Simulink Converter1/1 -> [dc_bus_terminal_current_inverter]  "idc"
  connections:
  h-mosfet/LConn1 -- uac_1(+)/RConn1
  h-mosfet/LConn2 -- uac_1(-)/RConn1
  h-mosfet/RConn2 -- Udc(-)/RConn1
  Current Sensor/LConn1 -- Udc(+)/RConn1
  h-mosfet/RConn1 -- Current Sensor/RConn2
  PS-Simulink Converter1/LConn1 -- Current Sensor/RConn1

== system battery_phfb_inv_single_phase/zvs_modA/dc//dc with galvanic isolation/stage-2 ==
  Current Sensor1 : fl_lib/Electrical/Electrical Sensors/Current Sensor
  PS-Simulink Converter2 : nesl_utility/PS-Simulink Converter  PhysicalDomain=network_engine_domain  SubClassName=ps_output  LeftPortType=input  RightPortType=output  PseudoPeriodic=off  Frequencies=[]  VectorFormat=1-D array  Unit=A  AffineConversion=on
  hf_trafo_center_tap : Subsystem  Commented=on
  hf_trafo_center_tap_ss : Subsystem
  hf_trafo_ideal : Subsystem  Commented=on
  hf_trafo_ss : Subsystem  Commented=on
  uac_1(+) : PMIOPort  Side=Left
  udc(+) : PMIOPort  Port=2  Side=Right
  uac_1(-) : PMIOPort  Port=3  Side=Left
  udc_(-) : PMIOPort  Port=4  Side=Right
  tag scope: LFu1_dc_current=global
  wires:
  PS-Simulink Converter2/1 -> [LFu1_dc_current]  "i_Ls"
  connections:
  Current Sensor1/RConn2 -- udc(+)/RConn1
  PS-Simulink Converter2/LConn1 -- Current Sensor1/RConn1
  hf_trafo_center_tap_ss/LConn1 -- uac_1(+)/RConn1
  hf_trafo_center_tap_ss/RConn1 -- Current Sensor1/LConn1
  hf_trafo_center_tap_ss/LConn2 -- uac_1(-)/RConn1
  hf_trafo_center_tap_ss/RConn2 -- udc_(-)/RConn1

== system battery_phfb_inv_single_phase/zvs_modA/zvs_ctrl/modulator1 ==
  phase_displacement : Inport
  Constant : Constant  Value=0.5
  Constant1 : Constant  Value=0
  Constant2 : Constant
  Gain : Gain  Gain=pi  OutDataTypeStr=double
  PWM generator 1 : Subsystem  mask{f=fPWM_ZVS, m_up=1, m_low=0, dead_time=dead_time, pos_cmd_gate=15, neg_cmd_gate=-10, polarity=1}
      mask prompts: f "Frequency (Hz)"; m_up "Max Input Modulation Value"; m_low "Min Input Modulation Value"; dead_time "Dead Time (s)"; pos_cmd_gate "Positive Gate Voltage (V)"; neg_cmd_gate "Negative Gate Voltage (V)"; polarity "Polarity (pu)"
  PWM generator 2 : Subsystem  mask{f=fPWM_ZVS, m_up=1, m_low=0, dead_time=dead_time, pos_cmd_gate=15, neg_cmd_gate=-10, polarity=1}
      mask prompts: f "Frequency (Hz)"; m_up "Max Input Modulation Value"; m_low "Min Input Modulation Value"; dead_time "Dead Time (s)"; pos_cmd_gate "Positive Gate Voltage (V)"; neg_cmd_gate "Negative Gate Voltage (V)"; polarity "Polarity (pu)"
  zvs_modulation : Scope  NumInputPorts=2
  gate_Q1 : Outport
  gate_Q2 : Outport  Port=2
  gate_Q3 : Outport  Port=3
  gate_Q4 : Outport  Port=4
  wires:
  PWM generator 2/2(m2) -> gate_Q4/1  "gate_Q4"
  PWM generator 2/1(m1) -> gate_Q3/1, zvs_modulation/2  "gate_Q3"
  PWM generator 1/2(m2) -> gate_Q2/1  "gate_Q2"
  PWM generator 1/1(m1) -> gate_Q1/1, zvs_modulation/1  "gate_Q1"
  phase_displacement/1 -> Gain/1
  Gain/1 -> PWM generator 2/2(phase)
  Constant/1 -> PWM generator 2/1(m_index), PWM generator 1/1(m_index)
  Constant1/1 -> PWM generator 1/2(phase)
  Constant2/1 -> PWM generator 2/3(polarity_input), PWM generator 1/3(polarity_input)

== system battery_phfb_inv_single_phase/zvs_modA/zvs_ctrl/references ==
  voltage_reference : Subsystem
  vout_ref : Outport
  wires:
  voltage_reference/1(vout_ref) -> vout_ref/1

== system battery_phfb_inv_single_phase/zvs_modA/zvs_ctrl/sampling_i_filter1 ==
  in : Inport
  1/Ti3 : Gain  Gain=1/I_FS  OutDataTypeStr=double  SaturateOnIntegerOverflow=on  ParamDataTypeStr=Inherit: Same as input
  Saturation : Saturate  UpperLimit=1  LowerLimit=0  OutDataTypeStr=double
  Zero-Order Hold2 : ZeroOrderHold  SampleTime=ts_zvs
  out_pu : Outport
  wires:
  in/1 -> 1/Ti3/1
  1/Ti3/1 -> Saturation/1
  Saturation/1 -> Zero-Order Hold2/1
  Zero-Order Hold2/1 -> out_pu/1

== system battery_phfb_inv_single_phase/zvs_modA/zvs_ctrl/sampling_v_filter1 ==
  in : Inport
  1/Ti3 : Gain  Gain=1/V_FS  OutDataTypeStr=double  SaturateOnIntegerOverflow=on  ParamDataTypeStr=Inherit: Same as input
  Saturation : Saturate  UpperLimit=1  LowerLimit=0  OutDataTypeStr=double
  Zero-Order Hold2 : ZeroOrderHold  SampleTime=ts_zvs
  out_pu : Outport
  wires:
  Zero-Order Hold2/1 -> out_pu/1
  1/Ti3/1 -> Saturation/1
  in/1 -> 1/Ti3/1
  Saturation/1 -> Zero-Order Hold2/1

== system battery_phfb_inv_single_phase/zvs_modA/zvs_ctrl/sampling_v_filter2 ==
  in : Inport
  1/Ti3 : Gain  Gain=1/V_FS  OutDataTypeStr=double  SaturateOnIntegerOverflow=on  ParamDataTypeStr=Inherit: Same as input
  Saturation : Saturate  UpperLimit=1  LowerLimit=0  OutDataTypeStr=double
  Zero-Order Hold2 : ZeroOrderHold  SampleTime=ts_zvs
  out_pu : Outport
  wires:
  in/1 -> 1/Ti3/1
  1/Ti3/1 -> Saturation/1
  Zero-Order Hold2/1 -> out_pu/1
  Saturation/1 -> Zero-Order Hold2/1

== system battery_phfb_inv_single_phase/zvs_modA/zvs_ctrl/vi ctrl ==
  iout : Inport
  vout : Inport  Port=2
  vout_ref : Inport  Port=3
  Constant : Constant  Value=Iout_dc_nom
  Iout Ctrl : Subsystem
  Min : MinMax  Inputs=2
  To Workspace1 : ToWorkspace  VariableName=phase_ctrl_out_modA_sim  SampleTime=ts_zvs
      settings: MaxDataPoints=Ns_zvs
  To Workspace2 : ToWorkspace  VariableName=pid_ctrlv_out_modA_sim  SampleTime=ts_zvs
      settings: MaxDataPoints=Ns_zvs
  To Workspace3 : ToWorkspace  VariableName=pid_ctrli_out_modA_sim  SampleTime=ts_zvs
      settings: MaxDataPoints=Ns_zvs
  Unit Delay2 : UnitDelay  SampleTime=ts_zvs  HasFrameUpgradeWarning=on
  Vout Ctrl : Subsystem
  zvs_ctrl : Scope  NumInputPorts=2
  phase_displacement : Outport
  wires:
  Unit Delay2/1 -> phase_displacement/1, To Workspace1/1
  iout/1 -> Iout Ctrl/2(iout)
  vout_ref/1 -> Vout Ctrl/1(vout_ref)
  vout/1 -> Vout Ctrl/2(vout)
  Vout Ctrl/1(ctrlv_out) -> zvs_ctrl/1, Unit Delay2/1, To Workspace2/1  "u_ctrl_out"
  Constant/1 -> Iout Ctrl/1(iout_ref)
  Iout Ctrl/1(ctrli_out) -> zvs_ctrl/2, To Workspace3/1, Min/2  "i_ctrl_out"

== system battery_phfb_inv_single_phase/inverter_modA/single phase inverter/HBridgeIdeal/switch_1 ==
  Current Sensor2 : fl_lib/Electrical/Electrical Sensors/Current Sensor
  Diode : fl_lib/Electrical/Electrical Elements/Diode  Vf=Vdon_diode V  Ron=Rdon_diode Ohm  Goff=1e-8 1/Ohm  i_specify=off  i_priority=None  i=0 A  i_nominal_specify=off  i_nominal_value=1  i_nominal_unit=A  v_specify=off  v_priority=None  v=0 V  v_nominal_specify=off  v_nominal_value=1  v_nominal_unit=V
  Switch : fl_lib/Electrical/Electrical Elements/Switch  R_closed=Ron Ohm  G_open=1e-8 1/Ohm  Threshold=7.5  i_specify=off  i_priority=None  i=0 A  i_nominal_specify=off  i_nominal_value=1  i_nominal_unit=A  v_specify=off  v_priority=None  v=0 V  v_nominal_specify=off  v_nominal_value=1  v_nominal_unit=V
  Voltage Sensor : fl_lib/Electrical/Electrical Sensors/Voltage Sensor
  iph2 : nesl_utility/PS-Simulink Converter  PhysicalDomain=network_engine_domain  SubClassName=ps_output  LeftPortType=input  RightPortType=output  PseudoPeriodic=off  Frequencies=[]  VectorFormat=1-D array  Unit=A  AffineConversion=off
  uph : nesl_utility/PS-Simulink Converter  PhysicalDomain=network_engine_domain  SubClassName=ps_output  LeftPortType=input  RightPortType=output  PseudoPeriodic=off  Frequencies=[]  VectorFormat=1-D array  Unit=V  AffineConversion=off
  G : PMIOPort  Side=Left
  C : PMIOPort  Port=2  Side=Left
  E : PMIOPort  Port=3  Side=Right
  tag scope: i_device_Q1_ideal_inv=global, u_device_Q1_ideal_inv=global
  wires:
  iph2/1 -> [i_device_Q1_ideal_inv]  "i_device_ideal_inv"
  uph/1 -> [u_device_Q1_ideal_inv]  "uph"
  connections:
  Switch/RConn2 -- Current Sensor2/RConn2 -- Voltage Sensor/LConn1 -- Diode/RConn1
  Switch/RConn1 -- G/RConn1
  Switch/LConn1 -- E/RConn1 -- Diode/LConn1 -- Voltage Sensor/RConn2
  Current Sensor2/LConn1 -- C/RConn1
  Current Sensor2/RConn1 -- iph2/LConn1
  Voltage Sensor/RConn1 -- uph/LConn1

== system battery_phfb_inv_single_phase/inverter_modA/single phase inverter/HBridgeIdeal/switch_2 ==
  Current Sensor2 : fl_lib/Electrical/Electrical Sensors/Current Sensor
  Diode : fl_lib/Electrical/Electrical Elements/Diode  Vf=Vdon_diode V  Ron=Rdon_diode Ohm  Goff=1e-8 1/Ohm  i_specify=off  i_priority=None  i=0 A  i_nominal_specify=off  i_nominal_value=1  i_nominal_unit=A  v_specify=off  v_priority=None  v=0 V  v_nominal_specify=off  v_nominal_value=1  v_nominal_unit=V
  Switch : fl_lib/Electrical/Electrical Elements/Switch  R_closed=Ron Ohm  G_open=1e-8 1/Ohm  Threshold=7.5  i_specify=off  i_priority=None  i=0 A  i_nominal_specify=off  i_nominal_value=1  i_nominal_unit=A  v_specify=off  v_priority=None  v=0 V  v_nominal_specify=off  v_nominal_value=1  v_nominal_unit=V
  Voltage Sensor : fl_lib/Electrical/Electrical Sensors/Voltage Sensor
  iph2 : nesl_utility/PS-Simulink Converter  PhysicalDomain=network_engine_domain  SubClassName=ps_output  LeftPortType=input  RightPortType=output  PseudoPeriodic=off  Frequencies=[]  VectorFormat=1-D array  Unit=A  AffineConversion=off
  uph : nesl_utility/PS-Simulink Converter  PhysicalDomain=network_engine_domain  SubClassName=ps_output  LeftPortType=input  RightPortType=output  PseudoPeriodic=off  Frequencies=[]  VectorFormat=1-D array  Unit=V  AffineConversion=off
  G : PMIOPort  Side=Left
  C : PMIOPort  Port=2  Side=Left
  E : PMIOPort  Port=3  Side=Right
  tag scope: i_device_Q2_ideal_inv=global, u_device_Q2_ideal_inv=global
  wires:
  uph/1 -> [u_device_Q2_ideal_inv]  "uph"
  iph2/1 -> [i_device_Q2_ideal_inv]  "i_device_ideal_inv"
  connections:
  E/RConn1 -- Switch/LConn1 -- Diode/LConn1 -- Voltage Sensor/RConn2
  Switch/RConn1 -- G/RConn1
  Switch/RConn2 -- Current Sensor2/RConn2 -- Voltage Sensor/LConn1 -- Diode/RConn1
  Voltage Sensor/RConn1 -- uph/LConn1
  Current Sensor2/RConn1 -- iph2/LConn1
  Current Sensor2/LConn1 -- C/RConn1

== system battery_phfb_inv_single_phase/inverter_modA/single phase inverter/HBridgeIdeal/switch_3 ==
  Diode : fl_lib/Electrical/Electrical Elements/Diode  Vf=Vdon_diode V  Ron=Rdon_diode Ohm  Goff=1e-8 1/Ohm  i_specify=off  i_priority=None  i=0 A  i_nominal_specify=off  i_nominal_value=1  i_nominal_unit=A  v_specify=off  v_priority=None  v=0 V  v_nominal_specify=off  v_nominal_value=1  v_nominal_unit=V
  Switch : fl_lib/Electrical/Electrical Elements/Switch  R_closed=Ron Ohm  G_open=1e-8 1/Ohm  Threshold=7.5  i_specify=off  i_priority=None  i=0 A  i_nominal_specify=off  i_nominal_value=1  i_nominal_unit=A  v_specify=off  v_priority=None  v=0 V  v_nominal_specify=off  v_nominal_value=1  v_nominal_unit=V
  G : PMIOPort  Side=Left
  C : PMIOPort  Port=2  Side=Left
  E : PMIOPort  Port=3  Side=Right
  connections:
  Switch/RConn2 -- C/RConn1 -- Diode/RConn1
  Switch/RConn1 -- G/RConn1
  Switch/LConn1 -- E/RConn1 -- Diode/LConn1

== system battery_phfb_inv_single_phase/inverter_modA/single phase inverter/HBridgeIdeal/switch_4 ==
  Diode : fl_lib/Electrical/Electrical Elements/Diode  Vf=Vdon_diode V  Ron=Rdon_diode Ohm  Goff=1e-8 1/Ohm  i_specify=off  i_priority=None  i=0 A  i_nominal_specify=off  i_nominal_value=1  i_nominal_unit=A  v_specify=off  v_priority=None  v=0 V  v_nominal_specify=off  v_nominal_value=1  v_nominal_unit=V
  Switch : fl_lib/Electrical/Electrical Elements/Switch  R_closed=Ron Ohm  G_open=1e-8 1/Ohm  Threshold=7.5  i_specify=off  i_priority=None  i=0 A  i_nominal_specify=off  i_nominal_value=1  i_nominal_unit=A  v_specify=off  v_priority=None  v=0 V  v_nominal_specify=off  v_nominal_value=1  v_nominal_unit=V
  G : PMIOPort  Side=Left
  C : PMIOPort  Port=2  Side=Left
  E : PMIOPort  Port=3  Side=Right
  connections:
  Diode/LConn1 -- E/RConn1 -- Switch/LConn1
  Switch/RConn1 -- G/RConn1
  Diode/RConn1 -- C/RConn1 -- Switch/RConn2

== system battery_phfb_inv_single_phase/inverter_modA/single phase inverter/HBridgeMosfet/mosfet_1 ==
  Current Sensor2 : fl_lib/Electrical/Electrical Sensors/Current Sensor
  MOSFET : ee_lib/Semiconductors & Converters/MOSFET (Ideal, Switching)  port_option=ee.enum.controlport.ps  Rds=Ron Ohm  Goff=1e-6 1/Ohm  Vth=7.5 V  diode_param=ee.enum.converters.protectiondiode.nodynamics  diode_Vf=Vgamma V  diode_Ron=0.001 Ohm  diode_Goff=1e-5 1/Ohm  diode_C=50e-9 F  diode_iRM=-235 A  diode_iF=300 A  diode_idot=-50 A/us  diode_trr_param=ee.enum.converters.diodeReverseParam.trr_factor  diode_trr_factor=3  diode_trr=15 us  diode_Qrr=1500 s*uA  ids_specify=off  ids_priority=None  ids=0 A  ids_nominal_specify=off  ids_nominal_value=1  ids_nominal_unit=A  vds_specify=off  vds_priority=None  vds=0 V  vds_nominal_specify=off  vds_nominal_value=1  vds_nominal_unit=V  vgs_specify=off  vgs_priority=None  vgs=0 V  vgs_nominal_specify=off  vgs_nominal_value=1  vgs_nominal_unit=V  thermal_loss_option=ee.enum.converters.thermalLossOption.constantvalues  Von_data=[0, 1.8, 3.2, 6, 10, 16; 0, 2, 5.5, 9.5, 15, 25] V  Tj=[298.15, 448.15] K  Iout_data=[0, 20, 40, 60, 80, 100] A  Eon_data=[0, 55.04, 124.57, 235.53, 362.12; 0, 71.25, 161.25, 304.88, 468.75] * 1e-6 J  Eoff_data=[0, 18, 30, 56.1, 76.5; 0, 22.5, 37.5, 70.13, 95.63] * 1e-6 J  Eon_data_3D=[zeros(2, 5, 3)] J  Eoff_data_3D=[zeros(2, 5, 3)] J  Tj_loss=[298.15, 448.15] K  Iout_data_loss=[0, 10, 20, 30, 40] A  tabulateWithVds=false  Vds_loss=[0, 150, 300] V  Eon_scalar=Eon J  Eoff_scalar=Eoff J  Voff=Voff_sw_losses V  Iout_scalar=Ion_sw_losses A  useCurrentFromPreviousCycle=true  useVoltageFromPreviousCycle=true  diodeModelType=ee.enum.converters.diodeModelType.pwl  diodeTableType=ee.enum.diode.tableType.IfMat  diode_ReverseIVType=ee.enum.diode.diodeReverseIV.constant  diode_IfMat=[.07, .12, .19, 1.75, 4.24, 7.32, 11.2; .16, .3, .72, 2.14, 4.02, 6.35, 9.12] A  diode_VfMat=[.9, 1.15, 1.25, 1.5, 1.75, 2.17, 2.6, 2.85; .58, .68, .75, 1.1, 1.38, 1.77, 2.27, 2.7] V  diode_TjVec=[25, 125] degC  diode_VfVec=[.5, .7, .9, 1.3, 1.7, 2.1, 2.5] V  diode_IfVec=[.1, .2, .5, 1, 2, 4, 7, 10] A  diode_IrMat=[1e-06, 2e-06, 5e-06, 1e-05, 2.5e-05, 5e-05, .0001; 2e-06, 5e-06, 1e-05, 4e-05, 8e-05, .0002, .0005] A  diode_VrMat=[10, 100, 200, 250, 300, 325, 350; 10, 70, 160, 220, 270, 300, 320] V  diode_VrVec=[10, 20, 40, 50, 70, 80, 100] V  diode_IrVec=[1e-06, 2e-06, 5e-06, 1e-05, 2e-05, 5e-05, .0001] A  diode_Vr=-600 V  diode_Ls=150 nH  diode_Erec=0.03 J  diode_rec_loss_model=ee.enum.diode.reverseRecoveryModel.fixed  diode_ErecVal=0 J  diode_scaleWithIandV=false  diode_ErecMat=zeros(2, 3) J  diode_TjrecVec=[298.15, 398.15] K  diode_IfrecVec=[.1, 1, 10] A  diode_IrecVal=10 A  diode_VrecVal=10 V  diode_tFilter=1 / 1000 / 100 s  separateThermalPortForDiode=false  thermal_network_parameterization=ee.enum.thermalNetworkTopology.external  Rth=[.03, .2] K/W  Rth_Cauer=[.03, .1, .2] K/W  Rth_Foster=[.03, .2] K/W  thermal_mass_parameterization=ee.enum.thermalNetwork.thermalmass  thermal_mass=[3, 25] J/K  thermal_mass_Cauer=[3, 10, 25] J/K  thermal_mass_Foster=[33, 50] J/K  thermal_time_constant=[.1, 5] s  thermal_time_constant_Cauer=[.1, 1, 5] s  thermal_time_constant_Foster=[1, 10] s  thermal_mass_initial_temperatures=[80, 80] degC  thermal_mass_initial_temperatures_Cauer=[25, 25, 25] degC  junction_thermal_mass=JunctionTermalMass J/K  Tvec_initial_Foster=[25, 25, 25, 25] degC  RthDiode=[.03, .2] K/W  RthCauerDiode=[.03, .1, .2] K/W  RthFosterDiode=[.03, .2] K/W  thermalMassDiode=[3, 25] J/K  thermalMassCauerDiode=[3, 10, 25] J/K  thermalMassFosterDiode=[33, 50] J/K  thermalTauDiode=[.1, 5] s  thermalTauCauerDiode=[.1, 1, 5] s  thermalTauFosterDiode=[1, 10] s  thermalMassInitTempDiode=[25, 25] degC  thermalMassInitTempCauerDiode=[25, 25, 25] degC  junctionthermalMassDiode=0.1 J/K  TVecInitialFosterDiode=[25, 25, 25, 25] degC  no_thermal_network=0  mosfet_junction_temperature_specify=on  mosfet_junction_temperature_priority=High  mosfet_junction_temperature=Tambient+DThs_init degC  mosfet_junction_temperature_nominal_specify=off  mosfet_junction_temperature_nominal_value=1  mosfet_junction_temperature_nominal_unit=degC  diode_junction_temperature_specify=off  diode_junction_temperature_priority=None  diode_junction_temperature=25 degC  diode_junction_temperature_nominal_specify=off  diode_junction_temperature_nominal_value=1  diode_junction_temperature_nominal_unit=degC  Qj_specify=off  Qj_priority=None  Qj=0 W  Qj_nominal_specify=off  Qj_nominal_value=1  Qj_nominal_unit=W  accumulatedSwitchingLosses_specify=off  accumulatedSwitchingLosses_priority=None  accumulatedSwitchingLosses=0 J
  Voltage Sensor : fl_lib/Electrical/Electrical Sensors/Voltage Sensor
  iph2 : nesl_utility/PS-Simulink Converter  PhysicalDomain=network_engine_domain  SubClassName=ps_output  LeftPortType=input  RightPortType=output  PseudoPeriodic=off  Frequencies=[]  VectorFormat=1-D array  Unit=A  AffineConversion=off
  uph : nesl_utility/PS-Simulink Converter  PhysicalDomain=network_engine_domain  SubClassName=ps_output  LeftPortType=input  RightPortType=output  PseudoPeriodic=off  Frequencies=[]  VectorFormat=1-D array  Unit=V  AffineConversion=off
  G : PMIOPort  Side=Left
  D : PMIOPort  Port=2  Side=Left
  S : PMIOPort  Port=3  Side=Right
  tag scope: i_device_Q1_mosfet_inv=global, u_device_Q1_mosfet_inv=global
  wires:
  iph2/1 -> [i_device_Q1_mosfet_inv]  "i_device_mosfet_inv"
  uph/1 -> [u_device_Q1_mosfet_inv]  "uph"
  connections:
  G/RConn1 -- MOSFET/LConn1
  MOSFET/RConn2 -- S/RConn1 -- Voltage Sensor/RConn2
  Current Sensor2/LConn1 -- D/RConn1
  Current Sensor2/RConn2 -- Voltage Sensor/LConn1 -- MOSFET/RConn1
  iph2/LConn1 -- Current Sensor2/RConn1
  Voltage Sensor/RConn1 -- uph/LConn1
